simulink model "Pitch_control"  (R2016a)
settings: Solver=VariableStepAuto  StartTime=0.0  StopTime=200.0  RelTol=1e-3
libraries: simulink_need_slupdate x1
settings Model: Creator=Jamie  LastModifiedBy=Jamie

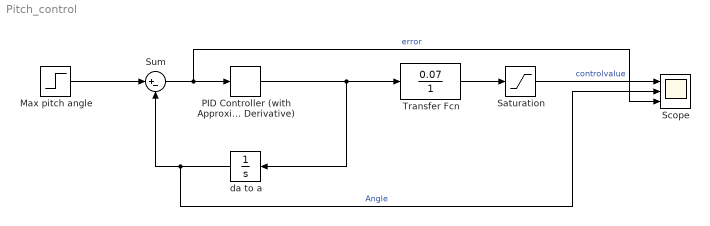
== system Pitch_control ==
  Max pitch angle : Step  After=-30  SampleTime=0
  PID Controller (with Approximate Derivative) : simulink_need_slupdate/PID Controller (with Approximate Derivative)  P=0.2  I=0  D=0  N=100
  Saturation : Saturate
  Scope : Scope  NumInputPorts=3
  Sum : Sum  Inputs=|+-
  Transfer Fcn : TransferFcn  Numerator=[0.07]  Denominator=[1]
  da to a : Integrator
  wires:
  Max pitch angle/1 -> Sum/1
  Sum/1 -> Scope/3, PID Controller (with Approximate Derivative)/1  "error"
  da to a/1 -> Sum/2, Scope/2  "Angle"
  PID Controller (with Approximate Derivative)/1 -> Transfer Fcn/1, da to a/1
  Transfer Fcn/1 -> Saturation/1
  Saturation/1 -> Scope/1  "controlvalue"
